simulink model "dynamictest"  (R2014a)
settings: Solver=ode45  StartTime=0.0  StopTime=15.0  RelTol=1e-3
settings Model: Creator=Think  LastModifiedBy=Think

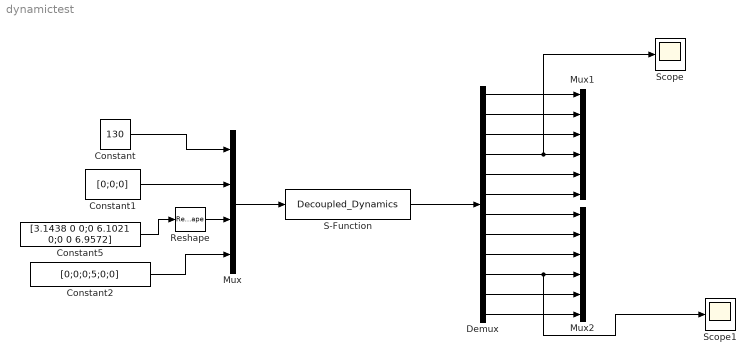
== system dynamictest ==
  Constant : Constant  Value=130
  Constant1 : Constant  Value=[0;0;0]
  Constant2 : Constant  Value=[0;0;0;5;0;0]  VectorParams1D=off
  Constant5 : Constant  Value=[3.1438 0 0;0 6.1021 0;0 0 6.9572]  VectorParams1D=off
  Demux : Demux  Outputs=12
  Mux : Mux
  Mux1 : Mux  Inputs=6
  Mux2 : Mux  Inputs=6
  Reshape : Reshape
  S-Function : S-Function  FunctionName=Decoupled_Dynamics  EnableBusSupport=off
  Scope : Scope
  Scope1 : Scope
  wires:
  Mux/1 -> S-Function/1
  S-Function/1 -> Demux/1
  Demux/1 -> Mux1/1
  Demux/2 -> Mux1/2
  Demux/3 -> Mux1/3
  Demux/4 -> Scope/1, Mux1/4
  Demux/5 -> Mux1/5
  Demux/6 -> Mux1/6
  Demux/7 -> Mux2/1
  Demux/8 -> Mux2/2
  Demux/9 -> Mux2/3
  Demux/10 -> Scope1/1, Mux2/4
  Demux/11 -> Mux2/5
  Demux/12 -> Mux2/6
  Constant/1 -> Mux/1
  Constant1/1 -> Mux/2
  Constant2/1 -> Mux/4
  Reshape/1 -> Mux/3
  Constant5/1 -> Reshape/1
